simulink model "MultilayerProcessControlSim"  (R2023b)
settings: Solver=ode4  StartTime=0.0  StopTime=10  RelTol=1e-3
undefined symbols (not defined in the file): DiscIntNeverNeededParam
libraries: dspstat3 x22, slpidlib x14
(part 1 of 3)
settings Model: Creator=yagiz  LastModifiedBy=yagiz

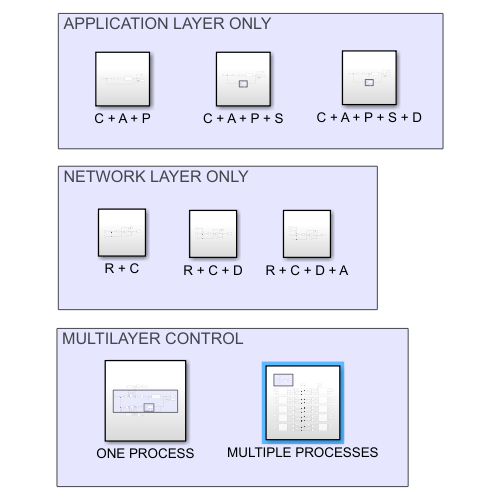
[thumbnail: Simulink's stored preview of the top-level diagram]
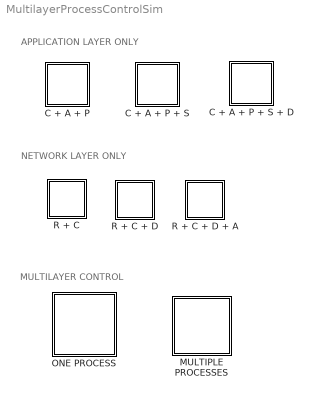
== system MultilayerProcessControlSim ==
  note: MULTILAYER CONTROL
  note: NETWORK LAYER ONLY
  note: APPLICATION LAYER ONLY
  C + A + P : Subsystem
  C + A + P + S : Subsystem
  C + A + P + S + D : Subsystem
  MULTIPLE PROCESSES : Subsystem
  ONE PROCESS : Subsystem
  R + C : Subsystem
  R + C + D : Subsystem
  R + C + D + A : Subsystem

== system MultilayerProcessControlSim/C + A + P ==
  ACTUATOR : Saturate  UpperLimit=150  LowerLimit=-150
  CONTROLLER : slpidlib/PID Controller  Controller=PI  Form=Parallel  TimeDomain=Continuous-time  UseExternalTs=off  SampleTime=-1  IntegratorMethod=Forward Euler  FilterMethod=Forward Euler  ControllerParametersSource=internal  P=1  I=3.6  UseKiTs=off  D=0  N=100  UseFilter=on  TunerSelectOption=Transfer Function Based (PID Tuner App)  InitialConditionSource=internal  InitialConditionForIntegrator=0  InitialConditionForFilter=0  DifferentiatorICPrevScaledInput=0  ExternalReset=none  TrackingMode=off  Kt=1  LimitOutput=off  SatLimitsSource=internal  UpperSaturationLimit=inf  LowerSaturationLimit=-inf  LinearizeAsGain=on  AntiWindupMode=none  Kb=1  LimitIntegrator=off  UpperIntegratorSaturationLimit=inf  LowerIntegratorSaturationLimit=-inf  POutMin=[]  POutMax=[]  IOutMin=[]  IOutMax=[]  DOutMin=[]  DOutMax=[]  NOutMin=[]  NOutMax=[]  SumOutMin=[]  SumOutMax=[]  SaturationOutMin=[]  SaturationOutMax=[]  PParamMin=[]  PParamMax=[]  IParamMin=[]  IParamMax=[]  DParamMin=[]  DParamMax=[]  NParamMin=[]  NParamMax=[]  KbParamMin=[]  KbParamMax=[]  KtParamMin=[]  KtParamMax=[]  KbOutMin=[]  KbOutMax=[]  KtOutMin=[]  KtOutMax=[]  IntegratorOutMin=[]  IntegratorOutMax=[]  FilterOutMin=[]  FilterOutMax=[]  SumI1OutMin=[]  SumI1OutMax=[]  SumI2OutMin=[]  SumI2OutMax=[]  SumI3OutMin=[]  SumI3OutMax=[]  SumI4OutMin=[]  SumI4OutMax=[]  SumDOutMin=[]  SumDOutMax=[]  DifferentiatorOutMin=[]  DifferentiatorOutMax=[]  FilterDiffOutCoefMin=[]  FilterDiffOutCoefMax=[]  ReciprocalOutMin=[]  ReciprocalOutMax=[]  SumDenOutMin=[]  SumDenOutMax=[]  SumNumOutMin=[]  SumNumOutMax=[]  DivideOutMin=[]  DivideOutMax=[]  UdiffTsProdOutMin=[]  UdiffTsProdOutMax=[]  NTsProdOutMin=[]  NTsProdOutMax=[]  UintegralTsProdOutMin=[]  UintegralTsProdOutMax=[]  UngainTsProdOutMin=[]  UngainTsProdOutMax=[]  ClampingZeroOutDataTypeStr=Inherit: Inherit via back propagation  ClampingZeroOutMin=[]  ClampingZeroOutMax=[]  FilterDenConstantOutDataTypeStr=Inherit: Inherit via back propagation  FilterDenConstantOutMin=[]  FilterDenConstantOutMax=[]  PCopyOutDataTypeStr=Inherit: Inherit via back propagation  PCopyOutMin=[]  PCopyOutMax=[]  NCopyOutDataTypeStr=Inherit: Inherit via back propagation  NCopyOutMin=[]  NCopyOutMax=[]  IntegratorContinuousStateAttributes=''  IntegratorStateMustResolveToSignalObject=off  IntegratorRTWStateStorageClass=Auto  FilterContinuousStateAttributes=''  FilterStateMustResolveToSignalObject=off  FilterRTWStateStorageClass=Auto  ParallelPVariant=InternalParameters  IdealPVariant=Disabled  IVariant=InternalParameters  DVariant=Disabled  IntegratorVariant=Continuous  SatVariant=Disabled  AWVariant=Passthrough  PCopyVariant=Disabled  TRVariant=Disabled  FdbkBlocksVariant=Forward  IdealPFdbkVariant=Disabled  SatFdbkVariant=Disabled  DerivativeFilterVariant=Disabled  NVariant=Disabled  NCopyVariant=Disabled_SignalSpec  FilterICVariant=Disabled  IntegratorICVariant=InternalICs  ExternalResetVariant=Disabled  TRSumVariant=Passthrough  SumFdbkVariant=Disabled  SumVariant=Sum_PI  TsampFilterVariant=InternalTs  TsampNgainVariant=Passthrough  TsampIntegralVariant=Disabled_SignalSpec  ExternalSaturationOutDataTypeStr=Inherit: Same as second input
  Constant3 : Constant  Value=20
  PROCESS : TransferFcn  Numerator=[1.38]  Denominator=[0.0007 0.1 0.00483]
  SETPOINT : Step  After=20  SampleTime=0
  Scope : Scope
  Sum : Sum  Inputs=|+-
  Sum4 : Sum  Inputs=|-+
  error : Display
  final value : Display
  wires:
  Sum/1 -> CONTROLLER/1
  CONTROLLER/1 -> ACTUATOR/1
  PROCESS/1 -> Sum4/1, Scope/1, final value/1, Sum/2  "output_app"
  Sum4/1 -> error/1
  SETPOINT/1 -> Sum/1
  Constant3/1 -> Sum4/2
  ACTUATOR/1 -> PROCESS/1

== system MultilayerProcessControlSim/C + A + P + S ==
  note: SENSOR
  ACTUATOR : Saturate  UpperLimit=150  LowerLimit=-150
  CONTROLLER : slpidlib/PID Controller  Controller=PI  Form=Parallel  TimeDomain=Continuous-time  UseExternalTs=off  SampleTime=-1  IntegratorMethod=Forward Euler  FilterMethod=Forward Euler  ControllerParametersSource=internal  P=1  I=3.6  UseKiTs=off  D=0  N=100  UseFilter=on  TunerSelectOption=Transfer Function Based (PID Tuner App)  InitialConditionSource=internal  InitialConditionForIntegrator=0  InitialConditionForFilter=0  DifferentiatorICPrevScaledInput=0  ExternalReset=none  TrackingMode=off  Kt=1  LimitOutput=off  SatLimitsSource=internal  UpperSaturationLimit=inf  LowerSaturationLimit=-inf  LinearizeAsGain=on  AntiWindupMode=none  Kb=1  LimitIntegrator=off  UpperIntegratorSaturationLimit=inf  LowerIntegratorSaturationLimit=-inf  POutMin=[]  POutMax=[]  IOutMin=[]  IOutMax=[]  DOutMin=[]  DOutMax=[]  NOutMin=[]  NOutMax=[]  SumOutMin=[]  SumOutMax=[]  SaturationOutMin=[]  SaturationOutMax=[]  PParamMin=[]  PParamMax=[]  IParamMin=[]  IParamMax=[]  DParamMin=[]  DParamMax=[]  NParamMin=[]  NParamMax=[]  KbParamMin=[]  KbParamMax=[]  KtParamMin=[]  KtParamMax=[]  KbOutMin=[]  KbOutMax=[]  KtOutMin=[]  KtOutMax=[]  IntegratorOutMin=[]  IntegratorOutMax=[]  FilterOutMin=[]  FilterOutMax=[]  SumI1OutMin=[]  SumI1OutMax=[]  SumI2OutMin=[]  SumI2OutMax=[]  SumI3OutMin=[]  SumI3OutMax=[]  SumI4OutMin=[]  SumI4OutMax=[]  SumDOutMin=[]  SumDOutMax=[]  DifferentiatorOutMin=[]  DifferentiatorOutMax=[]  FilterDiffOutCoefMin=[]  FilterDiffOutCoefMax=[]  ReciprocalOutMin=[]  ReciprocalOutMax=[]  SumDenOutMin=[]  SumDenOutMax=[]  SumNumOutMin=[]  SumNumOutMax=[]  DivideOutMin=[]  DivideOutMax=[]  UdiffTsProdOutMin=[]  UdiffTsProdOutMax=[]  NTsProdOutMin=[]  NTsProdOutMax=[]  UintegralTsProdOutMin=[]  UintegralTsProdOutMax=[]  UngainTsProdOutMin=[]  UngainTsProdOutMax=[]  ClampingZeroOutDataTypeStr=Inherit: Inherit via back propagation  ClampingZeroOutMin=[]  ClampingZeroOutMax=[]  FilterDenConstantOutDataTypeStr=Inherit: Inherit via back propagation  FilterDenConstantOutMin=[]  FilterDenConstantOutMax=[]  PCopyOutDataTypeStr=Inherit: Inherit via back propagation  PCopyOutMin=[]  PCopyOutMax=[]  NCopyOutDataTypeStr=Inherit: Inherit via back propagation  NCopyOutMin=[]  NCopyOutMax=[]  IntegratorContinuousStateAttributes=''  IntegratorStateMustResolveToSignalObject=off  IntegratorRTWStateStorageClass=Auto  FilterContinuousStateAttributes=''  FilterStateMustResolveToSignalObject=off  FilterRTWStateStorageClass=Auto  ParallelPVariant=InternalParameters  IdealPVariant=Disabled  IVariant=InternalParameters  DVariant=Disabled  IntegratorVariant=Continuous  SatVariant=Disabled  AWVariant=Passthrough  PCopyVariant=Disabled  TRVariant=Disabled  FdbkBlocksVariant=Forward  IdealPFdbkVariant=Disabled  SatFdbkVariant=Disabled  DerivativeFilterVariant=Disabled  NVariant=Disabled  NCopyVariant=Disabled_SignalSpec  FilterICVariant=Disabled  IntegratorICVariant=InternalICs  ExternalResetVariant=Disabled  TRSumVariant=Passthrough  SumFdbkVariant=Disabled  SumVariant=Sum_PI  TsampFilterVariant=InternalTs  TsampNgainVariant=Passthrough  TsampIntegralVariant=Disabled_SignalSpec  ExternalSaturationOutDataTypeStr=Inherit: Same as second input
  Constant3 : Constant  Value=20
  PROCESS : TransferFcn  Numerator=[1.38]  Denominator=[0.0007 0.1 0.00483]
  SETPOINT : Step  After=20  SampleTime=0
  Scope : Scope
  Sensor Accuracy : Sin  Amplitude=0.01  Bias=0.01  Frequency=50  SampleTime=0
  Sensor TF : TransferFcn  Denominator=[0.0002 1]
  Sum : Sum  Inputs=|+-
  Sum3 : Sum  Inputs=|++
  Sum4 : Sum  Inputs=|-+
  error : Display
  final value : Display
  wires:
  PROCESS/1 -> Sensor TF/1, Sum4/1, Scope/1, final value/1  "output_app"
  Sum/1 -> CONTROLLER/1
  CONTROLLER/1 -> ACTUATOR/1
  Constant3/1 -> Sum4/2
  Sum3/1 -> Sum/2
  ACTUATOR/1 -> PROCESS/1
  Sum4/1 -> error/1
  SETPOINT/1 -> Sum/1
  Sensor TF/1 -> Sum3/1
  Sensor Accuracy/1 -> Sum3/2

== system MultilayerProcessControlSim/C + A + P + S + D ==
  note: SENSOR
  ACTUATOR : Saturate  UpperLimit=150  LowerLimit=-150
  CONTROLLER : slpidlib/PID Controller  Controller=PI  Form=Parallel  TimeDomain=Continuous-time  UseExternalTs=off  SampleTime=-1  IntegratorMethod=Forward Euler  FilterMethod=Forward Euler  ControllerParametersSource=internal  P=1  I=3.6  UseKiTs=off  D=0  N=100  UseFilter=on  TunerSelectOption=Transfer Function Based (PID Tuner App)  InitialConditionSource=internal  InitialConditionForIntegrator=0  InitialConditionForFilter=0  DifferentiatorICPrevScaledInput=0  ExternalReset=none  TrackingMode=off  Kt=1  LimitOutput=off  SatLimitsSource=internal  UpperSaturationLimit=inf  LowerSaturationLimit=-inf  LinearizeAsGain=on  AntiWindupMode=none  Kb=1  LimitIntegrator=off  UpperIntegratorSaturationLimit=inf  LowerIntegratorSaturationLimit=-inf  POutMin=[]  POutMax=[]  IOutMin=[]  IOutMax=[]  DOutMin=[]  DOutMax=[]  NOutMin=[]  NOutMax=[]  SumOutMin=[]  SumOutMax=[]  SaturationOutMin=[]  SaturationOutMax=[]  PParamMin=[]  PParamMax=[]  IParamMin=[]  IParamMax=[]  DParamMin=[]  DParamMax=[]  NParamMin=[]  NParamMax=[]  KbParamMin=[]  KbParamMax=[]  KtParamMin=[]  KtParamMax=[]  KbOutMin=[]  KbOutMax=[]  KtOutMin=[]  KtOutMax=[]  IntegratorOutMin=[]  IntegratorOutMax=[]  FilterOutMin=[]  FilterOutMax=[]  SumI1OutMin=[]  SumI1OutMax=[]  SumI2OutMin=[]  SumI2OutMax=[]  SumI3OutMin=[]  SumI3OutMax=[]  SumI4OutMin=[]  SumI4OutMax=[]  SumDOutMin=[]  SumDOutMax=[]  DifferentiatorOutMin=[]  DifferentiatorOutMax=[]  FilterDiffOutCoefMin=[]  FilterDiffOutCoefMax=[]  ReciprocalOutMin=[]  ReciprocalOutMax=[]  SumDenOutMin=[]  SumDenOutMax=[]  SumNumOutMin=[]  SumNumOutMax=[]  DivideOutMin=[]  DivideOutMax=[]  UdiffTsProdOutMin=[]  UdiffTsProdOutMax=[]  NTsProdOutMin=[]  NTsProdOutMax=[]  UintegralTsProdOutMin=[]  UintegralTsProdOutMax=[]  UngainTsProdOutMin=[]  UngainTsProdOutMax=[]  ClampingZeroOutDataTypeStr=Inherit: Inherit via back propagation  ClampingZeroOutMin=[]  ClampingZeroOutMax=[]  FilterDenConstantOutDataTypeStr=Inherit: Inherit via back propagation  FilterDenConstantOutMin=[]  FilterDenConstantOutMax=[]  PCopyOutDataTypeStr=Inherit: Inherit via back propagation  PCopyOutMin=[]  PCopyOutMax=[]  NCopyOutDataTypeStr=Inherit: Inherit via back propagation  NCopyOutMin=[]  NCopyOutMax=[]  IntegratorContinuousStateAttributes=''  IntegratorStateMustResolveToSignalObject=off  IntegratorRTWStateStorageClass=Auto  FilterContinuousStateAttributes=''  FilterStateMustResolveToSignalObject=off  FilterRTWStateStorageClass=Auto  ParallelPVariant=InternalParameters  IdealPVariant=Disabled  IVariant=InternalParameters  DVariant=Disabled  IntegratorVariant=Continuous  SatVariant=Disabled  AWVariant=Passthrough  PCopyVariant=Disabled  TRVariant=Disabled  FdbkBlocksVariant=Forward  IdealPFdbkVariant=Disabled  SatFdbkVariant=Disabled  DerivativeFilterVariant=Disabled  NVariant=Disabled  NCopyVariant=Disabled_SignalSpec  FilterICVariant=Disabled  IntegratorICVariant=InternalICs  ExternalResetVariant=Disabled  TRSumVariant=Passthrough  SumFdbkVariant=Disabled  SumVariant=Sum_PI  TsampFilterVariant=InternalTs  TsampNgainVariant=Passthrough  TsampIntegralVariant=Disabled_SignalSpec  ExternalSaturationOutDataTypeStr=Inherit: Same as second input
  Constant3 : Constant  Value=20
  DISTURBANCE : Sin  Amplitude=0.1  Bias=0.1  Frequency=50  SampleTime=0
  PROCESS : TransferFcn  Numerator=[1.38]  Denominator=[0.0007 0.1 0.00483]
  SETPOINT : Step  After=20  SampleTime=0
  Scope : Scope
  Sensor Accuracy : Sin  Amplitude=0.01  Frequency=50  SampleTime=0
  Sensor TF : TransferFcn  Denominator=[0.0002 1]
  Sum : Sum  Inputs=|+-
  Sum2 : Sum  Inputs=|++
  Sum3 : Sum  Inputs=|++
  Sum4 : Sum  Inputs=|-+
  error : Display
  final value : Display
  wires:
  PROCESS/1 -> Sensor TF/1, Sum4/1, Scope/1, final value/1  "output_app"
  Sensor TF/1 -> Sum3/1
  Sensor Accuracy/1 -> Sum3/2
  Sum3/1 -> Sum/2
  CONTROLLER/1 -> ACTUATOR/1
  SETPOINT/1 -> Sum/1
  Sum4/1 -> error/1
  Constant3/1 -> Sum4/2
  Sum/1 -> CONTROLLER/1
  DISTURBANCE/1 -> Sum2/2
  ACTUATOR/1 -> Sum2/1
  Sum2/1 -> PROCESS/1

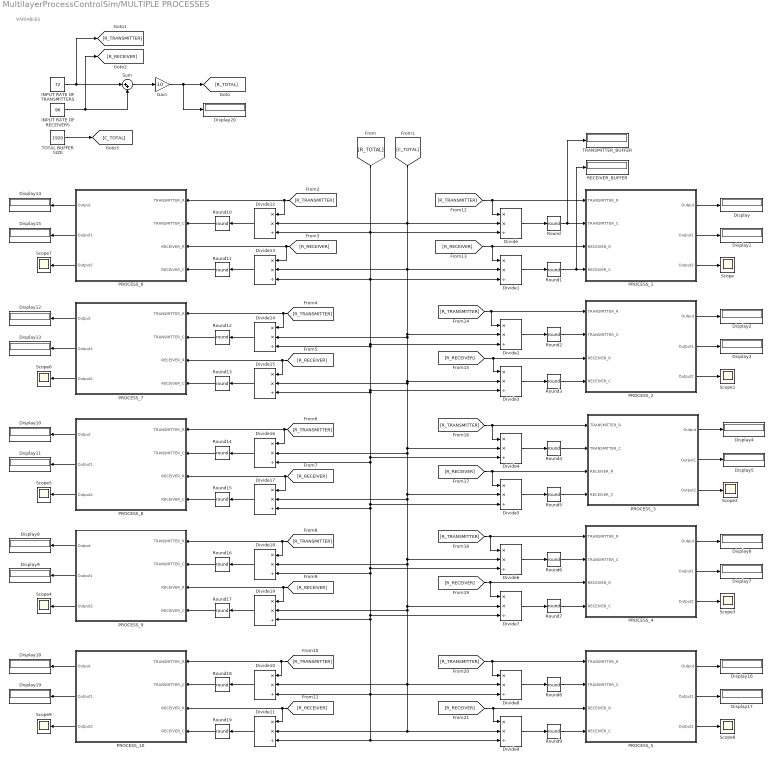
== system MultilayerProcessControlSim/MULTIPLE PROCESSES ==
  note: VARIABLES
  Display{,1..20} (21 alike) : Display
  Divide{,1..19} (20 alike) : Product  Inputs=**/
  Gain : Gain  Gain=10
  INPUT RATE OF RECEIVERS : Constant  Value=96
  INPUT RATE OF TRANSMITTERS : Constant  Value=72
  PROCESS_1 : Subsystem
  PROCESS_10 : Subsystem
  PROCESS_2 : Subsystem
  PROCESS_3 : Subsystem
  PROCESS_4 : Subsystem
  PROCESS_5 : Subsystem
  PROCESS_6 : Subsystem
  PROCESS_7 : Subsystem
  PROCESS_8 : Subsystem
  PROCESS_9 : Subsystem
  RECEIVER_BUFFER : Display
  Round{,1..19} (20 alike) : Rounding  Operator=round
  Scope{,1..9} (10 alike) : Scope
  Sum : Sum  Inputs=|++
  TOTAL BUFFER SIZE : Constant  Value=1920
  TRANSMITTER_BUFFER : Display
  wires:
  [C_TOTAL] -> Divide12/2, Divide13/2, Divide14/2, Divide15/2, Divide16/2, Divide17/2, Divide18/2, Divide19/2, Divide10/2, Divide8/2, Divide9/2, Divide11/2, Divide7/2, Divide6/2, Divide5/2, Divide4/2, Divide3/2, Divide2/2, Divide1/2, Divide/2
  Round2/1 -> PROCESS_2/2(TRANSMITTER_C)
  Round4/1 -> PROCESS_3/2(TRANSMITTER_C)
  [R_RECEIVER] -> Divide11/1, PROCESS_10/3(RECEIVER_R)
  Round17/1 -> PROCESS_9/4(RECEIVER_C)
  Round11/1 -> PROCESS_6/4(RECEIVER_C)
  PROCESS_5/2(Output1) -> Display17/1
  Divide6/1 -> Round6/1
  [R_TOTAL] -> Divide12/3, Divide13/3, Divide2/3, Divide14/3, Divide15/3, Divide16/3, Divide5/3, Divide17/3, Divide18/3, Divide19/3, Divide10/3, Divide11/3, Divide9/3, Divide8/3, Divide7/3, Divide6/3, Divide4/3, Divide3/3, Divide1/3, Divide/3
  Round12/1 -> PROCESS_7/2(TRANSMITTER_C)
  [R_RECEIVER] -> Divide1/1, PROCESS_1/3(RECEIVER_R)
  Round14/1 -> PROCESS_8/2(TRANSMITTER_C)
  Round10/1 -> PROCESS_6/2(TRANSMITTER_C)
  [R_TRANSMITTER] -> Divide10/1, PROCESS_10/1(TRANSMITTER_R)
  [R_RECEIVER] -> Divide13/1, PROCESS_6/3(RECEIVER_R)
  Divide17/1 -> Round15/1
  Divide11/1 -> Round19/1
  PROCESS_2/2(Output1) -> Display3/1
  [R_TRANSMITTER] -> Divide12/1, PROCESS_6/1(TRANSMITTER_R)
  PROCESS_6/1(Output) -> Display14/1
  Round3/1 -> PROCESS_2/4(RECEIVER_C)
  [R_RECEIVER] -> Divide5/1, PROCESS_3/3(RECEIVER_R)
  Round13/1 -> PROCESS_7/4(RECEIVER_C)
  Divide/1 -> Round/1
  [R_TRANSMITTER] -> Divide4/1, PROCESS_3/1(TRANSMITTER_R)
  [R_RECEIVER] -> Divide9/1, PROCESS_5/3(RECEIVER_R)
  Divide13/1 -> Round11/1
  PROCESS_2/3(Output2) -> Scope1/1
  [R_TRANSMITTER] -> Divide14/1, PROCESS_7/1(TRANSMITTER_R)
  [R_RECEIVER] -> Divide15/1, PROCESS_7/3(RECEIVER_R)
  PROCESS_10/1(Output) -> Display18/1
  [R_TRANSMITTER] -> Divide2/1, PROCESS_2/1(TRANSMITTER_R)
  Divide4/1 -> Round4/1
  PROCESS_1/1(Output) -> Display/1
  Round19/1 -> PROCESS_10/4(RECEIVER_C)
  PROCESS_9/1(Output) -> Display8/1
  PROCESS_2/1(Output) -> Display2/1
  PROCESS_10/3(Output2) -> Scope9/1
  Round9/1 -> PROCESS_5/4(RECEIVER_C)
  [R_TRANSMITTER] -> Divide6/1, PROCESS_4/1(TRANSMITTER_R)
  Divide9/1 -> Round9/1
  Round5/1 -> PROCESS_3/4(RECEIVER_C)
  PROCESS_10/2(Output1) -> Display19/1
  INPUT RATE OF TRANSMITTERS/1 -> [R_TRANSMITTER], Sum/1
  [R_TRANSMITTER] -> Divide8/1, PROCESS_5/1(TRANSMITTER_R)
  [R_RECEIVER] -> Divide17/1, PROCESS_8/3(RECEIVER_R)
  PROCESS_7/2(Output1) -> Display13/1
  Divide12/1 -> Round10/1
  Sum/1 -> Gain/1
  [R_TRANSMITTER] -> Divide18/1, PROCESS_9/1(TRANSMITTER_R)
  [R_TRANSMITTER] -> Divide16/1, PROCESS_8/1(TRANSMITTER_R)
  INPUT RATE OF RECEIVERS/1 -> Sum/2, [R_RECEIVER]
  [R_RECEIVER] -> Divide19/1, PROCESS_9/3(RECEIVER_R)
  PROCESS_5/1(Output) -> Display16/1
  Divide14/1 -> Round12/1
  PROCESS_7/1(Output) -> Display12/1
  PROCESS_3/3(Output2) -> Scope2/1
  Divide1/1 -> Round1/1
  Divide2/1 -> Round2/1
  Round15/1 -> PROCESS_8/4(RECEIVER_C)
  Divide3/1 -> Round3/1
  [R_RECEIVER] -> Divide3/1, PROCESS_2/3(RECEIVER_R)
  Round1/1 -> RECEIVER_BUFFER/1, PROCESS_1/4(RECEIVER_C)
  Divide19/1 -> Round17/1
  PROCESS_4/2(Output1) -> Display7/1
  Round18/1 -> PROCESS_10/2(TRANSMITTER_C)
  Gain/1 -> [R_TOTAL], Display20/1
  PROCESS_5/3(Output2) -> Scope8/1
  [R_TRANSMITTER] -> Divide/1, PROCESS_1/1(TRANSMITTER_R)
  PROCESS_1/3(Output2) -> Scope/1
  [R_RECEIVER] -> Divide7/1, PROCESS_4/3(RECEIVER_R)
  Divide10/1 -> Round18/1
  PROCESS_1/2(Output1) -> Display1/1
  PROCESS_4/1(Output) -> Display6/1
  Round16/1 -> PROCESS_9/2(TRANSMITTER_C)
  PROCESS_8/2(Output1) -> Display11/1
  Round/1 -> TRANSMITTER_BUFFER/1, PROCESS_1/2(TRANSMITTER_C)
  Round8/1 -> PROCESS_5/2(TRANSMITTER_C)
  PROCESS_7/3(Output2) -> Scope6/1
  PROCESS_6/3(Output2) -> Scope7/1
  PROCESS_6/2(Output1) -> Display15/1
  PROCESS_8/1(Output) -> Display10/1
  PROCESS_8/3(Output2) -> Scope5/1
  PROCESS_9/3(Output2) -> Scope4/1
  PROCESS_9/2(Output1) -> Display9/1
  Divide18/1 -> Round16/1
  PROCESS_3/2(Output1) -> Display5/1
  PROCESS_3/1(Output) -> Display4/1
  PROCESS_4/3(Output2) -> Scope3/1
  TOTAL BUFFER SIZE/1 -> [C_TOTAL]
  Round6/1 -> PROCESS_4/2(TRANSMITTER_C)
  Round7/1 -> PROCESS_4/4(RECEIVER_C)
  Divide7/1 -> Round7/1
  Divide5/1 -> Round5/1
  Divide16/1 -> Round14/1
  Divide8/1 -> Round8/1
  Divide15/1 -> Round13/1

== system MultilayerProcessControlSim/ONE PROCESS ==
  note: APPLICATION LAYER
  note: SENSOR
  ACTUATOR : Saturate  UpperLimit=150  LowerLimit=-150
  AVERAGE DELAY1 : Display
  AVERAGE DELAY2 : Display
  CONTROLLER : slpidlib/PID Controller  Controller=PI  Form=Parallel  TimeDomain=Continuous-time  UseExternalTs=off  SampleTime=-1  IntegratorMethod=Forward Euler  FilterMethod=Forward Euler  ControllerParametersSource=internal  P=1  I=3.6  UseKiTs=off  D=0  N=100  UseFilter=on  TunerSelectOption=Transfer Function Based (PID Tuner App)  InitialConditionSource=internal  InitialConditionForIntegrator=0  InitialConditionForFilter=0  DifferentiatorICPrevScaledInput=0  ExternalReset=none  TrackingMode=off  Kt=1  LimitOutput=off  SatLimitsSource=internal  UpperSaturationLimit=inf  LowerSaturationLimit=-inf  LinearizeAsGain=on  AntiWindupMode=none  Kb=1  LimitIntegrator=off  UpperIntegratorSaturationLimit=inf  LowerIntegratorSaturationLimit=-inf  POutMin=[]  POutMax=[]  IOutMin=[]  IOutMax=[]  DOutMin=[]  DOutMax=[]  NOutMin=[]  NOutMax=[]  SumOutMin=[]  SumOutMax=[]  SaturationOutMin=[]  SaturationOutMax=[]  PParamMin=[]  PParamMax=[]  IParamMin=[]  IParamMax=[]  DParamMin=[]  DParamMax=[]  NParamMin=[]  NParamMax=[]  KbParamMin=[]  KbParamMax=[]  KtParamMin=[]  KtParamMax=[]  KbOutMin=[]  KbOutMax=[]  KtOutMin=[]  KtOutMax=[]  IntegratorOutMin=[]  IntegratorOutMax=[]  FilterOutMin=[]  FilterOutMax=[]  SumI1OutMin=[]  SumI1OutMax=[]  SumI2OutMin=[]  SumI2OutMax=[]  SumI3OutMin=[]  SumI3OutMax=[]  SumI4OutMin=[]  SumI4OutMax=[]  SumDOutMin=[]  SumDOutMax=[]  DifferentiatorOutMin=[]  DifferentiatorOutMax=[]  FilterDiffOutCoefMin=[]  FilterDiffOutCoefMax=[]  ReciprocalOutMin=[]  ReciprocalOutMax=[]  SumDenOutMin=[]  SumDenOutMax=[]  SumNumOutMin=[]  SumNumOutMax=[]  DivideOutMin=[]  DivideOutMax=[]  UdiffTsProdOutMin=[]  UdiffTsProdOutMax=[]  NTsProdOutMin=[]  NTsProdOutMax=[]  UintegralTsProdOutMin=[]  UintegralTsProdOutMax=[]  UngainTsProdOutMin=[]  UngainTsProdOutMax=[]  ClampingZeroOutDataTypeStr=Inherit: Inherit via back propagation  ClampingZeroOutMin=[]  ClampingZeroOutMax=[]  FilterDenConstantOutDataTypeStr=Inherit: Inherit via back propagation  FilterDenConstantOutMin=[]  FilterDenConstantOutMax=[]  PCopyOutDataTypeStr=Inherit: Inherit via back propagation  PCopyOutMin=[]  PCopyOutMax=[]  NCopyOutDataTypeStr=Inherit: Inherit via back propagation  NCopyOutMin=[]  NCopyOutMax=[]  IntegratorContinuousStateAttributes=''  IntegratorStateMustResolveToSignalObject=off  IntegratorRTWStateStorageClass=Auto  FilterContinuousStateAttributes=''  FilterStateMustResolveToSignalObject=off  FilterRTWStateStorageClass=Auto  ParallelPVariant=InternalParameters  IdealPVariant=Disabled  IVariant=InternalParameters  DVariant=Disabled  IntegratorVariant=Continuous  SatVariant=Disabled  AWVariant=Passthrough  PCopyVariant=Disabled  TRVariant=Disabled  FdbkBlocksVariant=Forward  IdealPFdbkVariant=Disabled  SatFdbkVariant=Disabled  DerivativeFilterVariant=Disabled  NVariant=Disabled  NCopyVariant=Disabled_SignalSpec  FilterICVariant=Disabled  IntegratorICVariant=InternalICs  ExternalResetVariant=Disabled  TRSumVariant=Passthrough  SumFdbkVariant=Disabled  SumVariant=Sum_PI  TsampFilterVariant=InternalTs  TsampNgainVariant=Passthrough  TsampIntegralVariant=Disabled_SignalSpec  ExternalSaturationOutDataTypeStr=Inherit: Same as second input
  Constant3 : Constant  Value=20
  DISTURBANCE : Sin  Amplitude=0.1  Bias=0.05  Frequency=50  SampleTime=0
  DRIVER-PLC NETWORK : Subsystem
  Memory : Memory
  Memory1 : Memory
  Moving Average : dspstat3/Moving Average  Method=Sliding window  ForgettingFactorPort=off  SpecifyWindowLength=on  WindowLength=4  OverlapLength=3  AllowArbitraryInputLength=off  ForgettingFactor=0.9  SimulateUsing=Code generation
  Moving Average1 : dspstat3/Moving Average  Method=Sliding window  ForgettingFactorPort=off  SpecifyWindowLength=on  WindowLength=4  OverlapLength=3  AllowArbitraryInputLength=off  ForgettingFactor=0.9  SimulateUsing=Code generation
  PLC-DRIVER NETWORK : Subsystem
  PROCESS : TransferFcn  Numerator=[1.38]  Denominator=[0.0007 0.1 0.00483]
  SETPOINT : Step  After=20  SampleTime=0
  Scope1 : Scope  NumInputPorts=2
  Sensor Accuracy : Sin  Amplitude=0.01  Frequency=50  SampleTime=0
  Sensor TF : TransferFcn  Denominator=[0.0002 1]
  Sum : Sum  Inputs=|+-
  Sum2 : Sum  Inputs=|++
  Sum3 : Sum  Inputs=|++
  Sum4 : Sum  Inputs=|-+
  Switch : Switch  Criteria=u2 > Threshold  Threshold=9600  SaturateOnIntegerOverflow=off  InputSameDT=off
  Switch1 : Switch  Criteria=u2 > Threshold  Threshold=9600  SaturateOnIntegerOverflow=off  InputSameDT=off
  Variable Time Delay : VariableTransportDelay  MaximumDelay=10
  Variable Time Delay1 : VariableTransportDelay  MaximumDelay=10
  error : Display
  final value : Display
  wires:
  Moving Average1/1 -> AVERAGE DELAY1/1
  Sum2/1 -> PROCESS/1
  Moving Average/1 -> AVERAGE DELAY2/1
  Switch1/1 -> Memory1/1, Variable Time Delay1/1
  Variable Time Delay/1 -> ACTUATOR/1
  DRIVER-PLC NETWORK/2(DELAY1) -> Variable Time Delay1/2, Moving Average/1
  Sum/1 -> CONTROLLER/1
  PROCESS/1 -> final value/1, Sum4/1, Scope1/2, Sensor TF/1  "output_app"
  DRIVER-PLC NETWORK/1(Q) -> Switch1/2
  PLC-DRIVER NETWORK/1(DELAY1) -> Moving Average1/1, Variable Time Delay/2
  SETPOINT/1 -> Sum/1
  PLC-DRIVER NETWORK/2(Q) -> Switch/2
  Sensor TF/1 -> Sum3/1
  Constant3/1 -> Sum4/2
  Sensor Accuracy/1 -> Sum3/2
  Sum4/1 -> error/1
  Switch/1 -> Memory/1, Variable Time Delay/1
  Variable Time Delay1/1 -> Sum/2, Scope1/1  "feedback_out"
  CONTROLLER/1 -> Switch/3
  Memory1/1 -> Switch1/1
  DISTURBANCE/1 -> Sum2/2
  ACTUATOR/1 -> Sum2/1
  Memory/1 -> Switch/1
  Sum3/1 -> Switch1/3

== system MultilayerProcessControlSim/R + C ==
  BUFFER : Constant  Value=96
  Discrete-Time Integrator1 : DiscreteIntegrator  SampleTime=-1  LimitOutput=on  UpperSaturationLimit=9600  LowerSaturationLimit=0  ICPrevOutput=DiscIntNeverNeededParam  ICPrevScaledInput=DiscIntNeverNeededParam
  Divide1 : Product  Inputs=*/
  INPUT RATE : Constant  Value=72
  Network Delay : Display
  PROPAGATION DELAY : Constant  Value=0.01
  Scope : Scope  NumInputPorts=2
  Sum1 : Sum  Inputs=|++
  Sum2 : Sum  Inputs=|+-
  wires:
  PROPAGATION DELAY/1 -> Sum1/2  "TAU_P"
  BUFFER/1 -> Divide1/2, Sum2/2
  Divide1/1 -> Sum1/1, Scope/2  "TAU_Q"
  Discrete-Time Integrator1/1 -> Scope/1, Divide1/1  "Q"
  INPUT RATE/1 -> Sum2/1
  Sum1/1 -> Network Delay/1  "DELAY"
  Sum2/1 -> Discrete-Time Integrator1/1  "Q_dot"

== system MultilayerProcessControlSim/R + C + D ==
  BUFFER : Constant  Value=96
  DISTURBANCE : DiscretePulseGenerator  PulseType=Time based  Amplitude=48  Period=0.01  PulseWidth=50
  Discrete-Time Integrator1 : DiscreteIntegrator  SampleTime=-1  LimitOutput=on  UpperSaturationLimit=9600  LowerSaturationLimit=0  ICPrevOutput=DiscIntNeverNeededParam  ICPrevScaledInput=DiscIntNeverNeededParam
  Divide1 : Product  Inputs=*/
  INPUT RATE : Constant  Value=72
  Network Delay : Display
  PROPAGATION DELAY : Constant  Value=0.01
  Scope : Scope  NumInputPorts=2
  Sum : Sum  Inputs=+|+|-
  Sum1 : Sum  Inputs=|++
  wires:
  BUFFER/1 -> Sum/3, Divide1/2
  Divide1/1 -> Sum1/1, Scope/2  "TAU_Q"
  INPUT RATE/1 -> Sum/2
  DISTURBANCE/1 -> Sum/1
  Sum1/1 -> Network Delay/1  "DELAY"
  PROPAGATION DELAY/1 -> Sum1/2  "TAU_P"
  Discrete-Time Integrator1/1 -> Scope/1, Divide1/1  "Q"
  Sum/1 -> Discrete-Time Integrator1/1  "Q_dot"

== system MultilayerProcessControlSim/R + C + D + A ==
  ATTACK : Constant  Value=10000
  BUFFER : Constant  Value=96
  DISTURBANCE : DiscretePulseGenerator  PulseType=Time based  Amplitude=24  Period=0.001  PulseWidth=50
  Discrete-Time Integrator1 : DiscreteIntegrator  SampleTime=-1  LimitOutput=on  UpperSaturationLimit=9600  LowerSaturationLimit=0  ICPrevOutput=DiscIntNeverNeededParam  ICPrevScaledInput=DiscIntNeverNeededParam
  Divide1 : Product  Inputs=*/
  INPUT RATE : Constant  Value=72
  Network Delay : Display
  PROPAGATION DELAY : Constant  Value=0.01
  Scope : Scope  NumInputPorts=2
  Sum : Sum  Inputs=++|+|-
  Sum1 : Sum  Inputs=|++
  wires:
  Divide1/1 -> Sum1/1, Scope/2  "TAU_Q"
  PROPAGATION DELAY/1 -> Sum1/2  "TAU_P"
  Sum1/1 -> Network Delay/1  "DELAY"
  Sum/1 -> Discrete-Time Integrator1/1  "Q_dot"
  Discrete-Time Integrator1/1 -> Scope/1, Divide1/1  "Q"
  BUFFER/1 -> Sum/4, Divide1/2
  INPUT RATE/1 -> Sum/3
  DISTURBANCE/1 -> Sum/2
  ATTACK/1 -> Sum/1

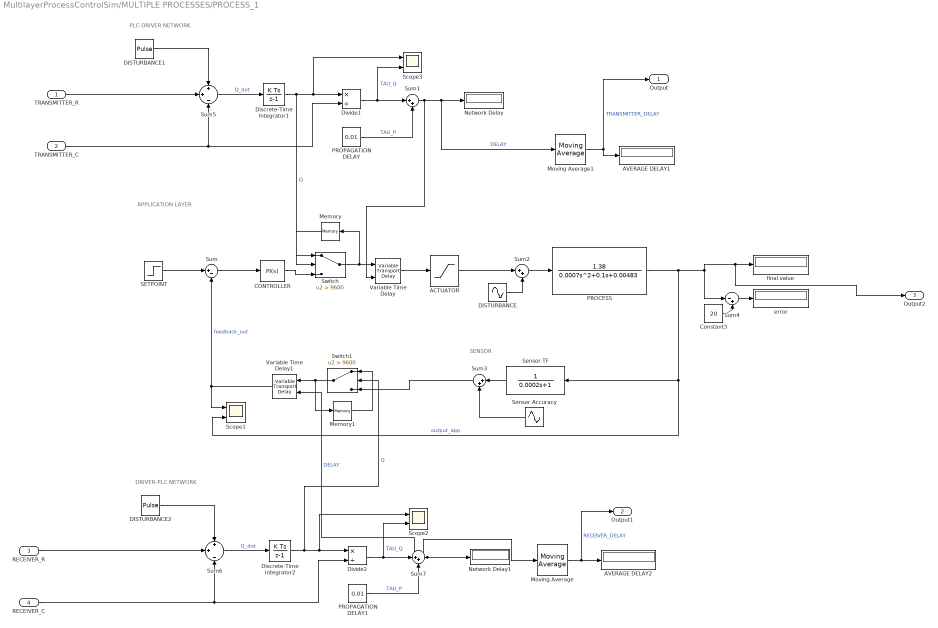
== system MultilayerProcessControlSim/MULTIPLE PROCESSES/PROCESS_1 ==
  note: DRIVER-PLC NETWORK
  note: PLC-DRIVER NETWORK
  note: APPLICATION LAYER
  note: SENSOR
  TRANSMITTER_R : Inport
  TRANSMITTER_C : Inport  Port=2
  RECEIVER_R : Inport  Port=3
  RECEIVER_C : Inport  Port=4
  ACTUATOR : Saturate  UpperLimit=150  LowerLimit=-150
  AVERAGE DELAY1 : Display
  AVERAGE DELAY2 : Display
  CONTROLLER : slpidlib/PID Controller  Controller=PI  Form=Parallel  TimeDomain=Continuous-time  UseExternalTs=off  SampleTime=-1  IntegratorMethod=Forward Euler  FilterMethod=Forward Euler  ControllerParametersSource=internal  P=1  I=3.6  UseKiTs=off  D=0  N=100  UseFilter=on  TunerSelectOption=Transfer Function Based (PID Tuner App)  InitialConditionSource=internal  InitialConditionForIntegrator=0  InitialConditionForFilter=0  DifferentiatorICPrevScaledInput=0  ExternalReset=none  TrackingMode=off  Kt=1  LimitOutput=off  SatLimitsSource=internal  UpperSaturationLimit=inf  LowerSaturationLimit=-inf  LinearizeAsGain=on  AntiWindupMode=none  Kb=1  LimitIntegrator=off  UpperIntegratorSaturationLimit=inf  LowerIntegratorSaturationLimit=-inf  POutMin=[]  POutMax=[]  IOutMin=[]  IOutMax=[]  DOutMin=[]  DOutMax=[]  NOutMin=[]  NOutMax=[]  SumOutMin=[]  SumOutMax=[]  SaturationOutMin=[]  SaturationOutMax=[]  PParamMin=[]  PParamMax=[]  IParamMin=[]  IParamMax=[]  DParamMin=[]  DParamMax=[]  NParamMin=[]  NParamMax=[]  KbParamMin=[]  KbParamMax=[]  KtParamMin=[]  KtParamMax=[]  KbOutMin=[]  KbOutMax=[]  KtOutMin=[]  KtOutMax=[]  IntegratorOutMin=[]  IntegratorOutMax=[]  FilterOutMin=[]  FilterOutMax=[]  SumI1OutMin=[]  SumI1OutMax=[]  SumI2OutMin=[]  SumI2OutMax=[]  SumI3OutMin=[]  SumI3OutMax=[]  SumI4OutMin=[]  SumI4OutMax=[]  SumDOutMin=[]  SumDOutMax=[]  DifferentiatorOutMin=[]  DifferentiatorOutMax=[]  FilterDiffOutCoefMin=[]  FilterDiffOutCoefMax=[]  ReciprocalOutMin=[]  ReciprocalOutMax=[]  SumDenOutMin=[]  SumDenOutMax=[]  SumNumOutMin=[]  SumNumOutMax=[]  DivideOutMin=[]  DivideOutMax=[]  UdiffTsProdOutMin=[]  UdiffTsProdOutMax=[]  NTsProdOutMin=[]  NTsProdOutMax=[]  UintegralTsProdOutMin=[]  UintegralTsProdOutMax=[]  UngainTsProdOutMin=[]  UngainTsProdOutMax=[]  ClampingZeroOutDataTypeStr=Inherit: Inherit via back propagation  ClampingZeroOutMin=[]  ClampingZeroOutMax=[]  FilterDenConstantOutDataTypeStr=Inherit: Inherit via back propagation  FilterDenConstantOutMin=[]  FilterDenConstantOutMax=[]  PCopyOutDataTypeStr=Inherit: Inherit via back propagation  PCopyOutMin=[]  PCopyOutMax=[]  NCopyOutDataTypeStr=Inherit: Inherit via back propagation  NCopyOutMin=[]  NCopyOutMax=[]  IntegratorContinuousStateAttributes=''  IntegratorStateMustResolveToSignalObject=off  IntegratorRTWStateStorageClass=Auto  FilterContinuousStateAttributes=''  FilterStateMustResolveToSignalObject=off  FilterRTWStateStorageClass=Auto  ParallelPVariant=InternalParameters  IdealPVariant=Disabled  IVariant=InternalParameters  DVariant=Disabled  IntegratorVariant=Continuous  SatVariant=Disabled  AWVariant=Passthrough  PCopyVariant=Disabled  TRVariant=Disabled  FdbkBlocksVariant=Forward  IdealPFdbkVariant=Disabled  SatFdbkVariant=Disabled  DerivativeFilterVariant=Disabled  NVariant=Disabled  NCopyVariant=Disabled_SignalSpec  FilterICVariant=Disabled  IntegratorICVariant=InternalICs  ExternalResetVariant=Disabled  TRSumVariant=Passthrough  SumFdbkVariant=Disabled  SumVariant=Sum_PI  TsampFilterVariant=InternalTs  TsampNgainVariant=Passthrough  TsampIntegralVariant=Disabled_SignalSpec  ExternalSaturationOutDataTypeStr=Inherit: Same as second input
  Constant3 : Constant  Value=20
  DISTURBANCE : Sin  Amplitude=0.1  Bias=0.05  Frequency=50  SampleTime=0
  DISTURBANCE1 : DiscretePulseGenerator  PulseType=Time based  Amplitude=0  Period=0.001  PulseWidth=50
  DISTURBANCE2 : DiscretePulseGenerator  PulseType=Time based  Amplitude=0  Period=0.001  PulseWidth=50
  Discrete-Time Integrator1 : DiscreteIntegrator  SampleTime=-1  LimitOutput=on  UpperSaturationLimit=9600  LowerSaturationLimit=0  ICPrevOutput=DiscIntNeverNeededParam  ICPrevScaledInput=DiscIntNeverNeededParam
  Discrete-Time Integrator2 : DiscreteIntegrator  SampleTime=-1  LimitOutput=on  UpperSaturationLimit=9600  LowerSaturationLimit=0  ICPrevOutput=DiscIntNeverNeededParam  ICPrevScaledInput=DiscIntNeverNeededParam
  Divide1 : Product  Inputs=*/
  Divide2 : Product  Inputs=*/
  Memory : Memory
  Memory1 : Memory
  Moving Average : dspstat3/Moving Average  Method=Sliding window  ForgettingFactorPort=off  SpecifyWindowLength=on  WindowLength=4  OverlapLength=3  AllowArbitraryInputLength=off  ForgettingFactor=0.9  SimulateUsing=Code generation
  Moving Average1 : dspstat3/Moving Average  Method=Sliding window  ForgettingFactorPort=off  SpecifyWindowLength=on  WindowLength=4  OverlapLength=3  AllowArbitraryInputLength=off  ForgettingFactor=0.9  SimulateUsing=Code generation
  Network Delay : Display
  Network Delay1 : Display
  PROCESS : TransferFcn  Numerator=[1.38]  Denominator=[0.0007 0.1 0.00483]
  PROPAGATION DELAY : Constant  Value=0.01
  PROPAGATION DELAY1 : Constant  Value=0.01
  SETPOINT : Step  After=20  SampleTime=0
  Scope1 : Scope  NumInputPorts=2
  Scope2 : Scope  NumInputPorts=2
  Scope3 : Scope  NumInputPorts=2
  Sensor Accuracy : Sin  Amplitude=0.01  Frequency=50  SampleTime=0
  Sensor TF : TransferFcn  Denominator=[0.0002 1]
  Sum : Sum  Inputs=|+-
  Sum{1..3,7} (4 alike) : Sum  Inputs=|++
  Sum4 : Sum  Inputs=|-+
  Sum5 : Sum  Inputs=+|+|-
  Sum6 : Sum  Inputs=+|+|-
  Switch : Switch  Criteria=u2 > Threshold  Threshold=9600  SaturateOnIntegerOverflow=off  InputSameDT=off
  Switch1 : Switch  Criteria=u2 > Threshold  Threshold=9600  SaturateOnIntegerOverflow=off  InputSameDT=off
  Variable Time Delay : VariableTransportDelay  MaximumDelay=10
  Variable Time Delay1 : VariableTransportDelay  MaximumDelay=10
  error : Display
  final value : Display
  Output : Outport
  Output1 : Outport  Port=2
  Output2 : Outport  Port=3
  wires:
  RECEIVER_C/1 -> Sum6/3, Divide2/2
  DISTURBANCE1/1 -> Sum5/1
  Sum1/1 -> Moving Average1/1, Network Delay/1, Variable Time Delay/2  "DELAY"
  TRANSMITTER_C/1 -> Divide1/2, Sum5/3
  CONTROLLER/1 -> Switch/3
  Sum3/1 -> Switch1/3
  Moving Average1/1 -> Output/1, AVERAGE DELAY1/1  "TRANSMITTER_DELAY"
  Memory1/1 -> Switch1/1
  Memory/1 -> Switch/1
  Switch/1 -> Memory/1, Variable Time Delay/1
  TRANSMITTER_R/1 -> Sum5/2
  ACTUATOR/1 -> Sum2/1
  RECEIVER_R/1 -> Sum6/2
  SETPOINT/1 -> Sum/1
  Sum7/1 -> Variable Time Delay1/2, Moving Average/1, Network Delay1/1  "DELAY"
  Discrete-Time Integrator2/1 -> Switch1/2, Scope2/1, Divide2/1  "Q"
  Switch1/1 -> Memory1/1, Variable Time Delay1/1
  DISTURBANCE2/1 -> Sum6/1
  Variable Time Delay1/1 -> Sum/2, Scope1/1  "feedback_out"
  Discrete-Time Integrator1/1 -> Scope3/1, Divide1/1, Switch/2  "Q"
  Divide2/1 -> Sum7/1, Scope2/2  "TAU_Q"
  Moving Average/1 -> Output1/1, AVERAGE DELAY2/1  "RECEIVER_DELAY"
  Divide1/1 -> Scope3/2, Sum1/1  "TAU_Q"
  Sensor Accuracy/1 -> Sum3/2
  Sum6/1 -> Discrete-Time Integrator2/1  "Q_dot"
  PROCESS/1 -> Output2/1, final value/1, Sum4/1, Sensor TF/1, Scope1/2  "output_app"
  PROPAGATION DELAY1/1 -> Sum7/2  "TAU_P"
  Sum5/1 -> Discrete-Time Integrator1/1  "Q_dot"
  Sum2/1 -> PROCESS/1
  Sensor TF/1 -> Sum3/1
  PROPAGATION DELAY/1 -> Sum1/2  "TAU_P"
  Variable Time Delay/1 -> ACTUATOR/1
  Sum4/1 -> error/1
  Constant3/1 -> Sum4/2
  DISTURBANCE/1 -> Sum2/2
  Sum/1 -> CONTROLLER/1

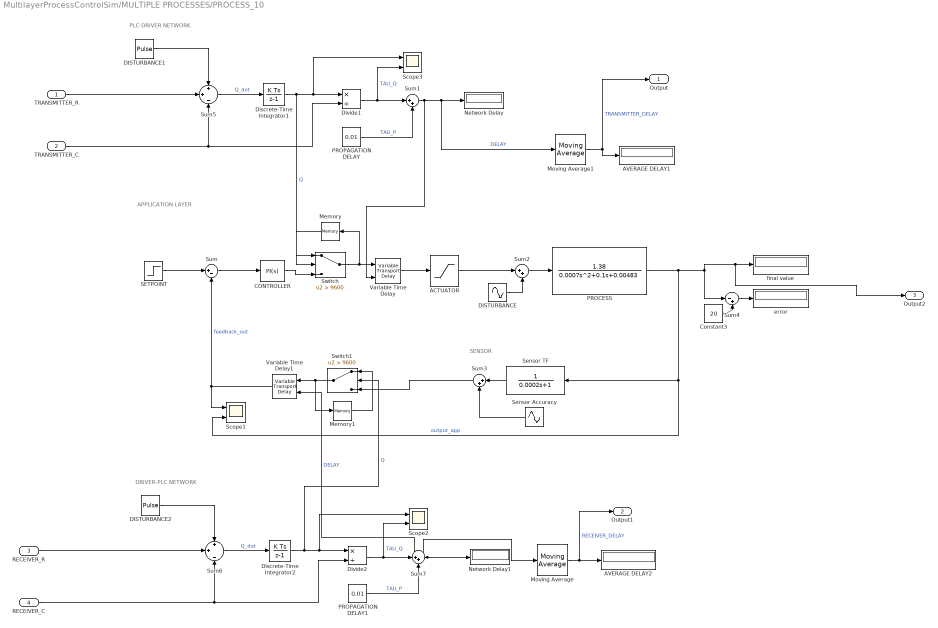
== system MultilayerProcessControlSim/MULTIPLE PROCESSES/PROCESS_10 ==
  note: DRIVER-PLC NETWORK
  note: PLC-DRIVER NETWORK
  note: APPLICATION LAYER
  note: SENSOR
  TRANSMITTER_R : Inport
  TRANSMITTER_C : Inport  Port=2
  RECEIVER_R : Inport  Port=3
  RECEIVER_C : Inport  Port=4
  ACTUATOR : Saturate  UpperLimit=150  LowerLimit=-150
  AVERAGE DELAY1 : Display
  AVERAGE DELAY2 : Display
  CONTROLLER : slpidlib/PID Controller  Controller=PI  Form=Parallel  TimeDomain=Continuous-time  UseExternalTs=off  SampleTime=-1  IntegratorMethod=Forward Euler  FilterMethod=Forward Euler  ControllerParametersSource=internal  P=1  I=3.6  UseKiTs=off  D=0  N=100  UseFilter=on  TunerSelectOption=Transfer Function Based (PID Tuner App)  InitialConditionSource=internal  InitialConditionForIntegrator=0  InitialConditionForFilter=0  DifferentiatorICPrevScaledInput=0  ExternalReset=none  TrackingMode=off  Kt=1  LimitOutput=off  SatLimitsSource=internal  UpperSaturationLimit=inf  LowerSaturationLimit=-inf  LinearizeAsGain=on  AntiWindupMode=none  Kb=1  LimitIntegrator=off  UpperIntegratorSaturationLimit=inf  LowerIntegratorSaturationLimit=-inf  POutMin=[]  POutMax=[]  IOutMin=[]  IOutMax=[]  DOutMin=[]  DOutMax=[]  NOutMin=[]  NOutMax=[]  SumOutMin=[]  SumOutMax=[]  SaturationOutMin=[]  SaturationOutMax=[]  PParamMin=[]  PParamMax=[]  IParamMin=[]  IParamMax=[]  DParamMin=[]  DParamMax=[]  NParamMin=[]  NParamMax=[]  KbParamMin=[]  KbParamMax=[]  KtParamMin=[]  KtParamMax=[]  KbOutMin=[]  KbOutMax=[]  KtOutMin=[]  KtOutMax=[]  IntegratorOutMin=[]  IntegratorOutMax=[]  FilterOutMin=[]  FilterOutMax=[]  SumI1OutMin=[]  SumI1OutMax=[]  SumI2OutMin=[]  SumI2OutMax=[]  SumI3OutMin=[]  SumI3OutMax=[]  SumI4OutMin=[]  SumI4OutMax=[]  SumDOutMin=[]  SumDOutMax=[]  DifferentiatorOutMin=[]  DifferentiatorOutMax=[]  FilterDiffOutCoefMin=[]  FilterDiffOutCoefMax=[]  ReciprocalOutMin=[]  ReciprocalOutMax=[]  SumDenOutMin=[]  SumDenOutMax=[]  SumNumOutMin=[]  SumNumOutMax=[]  DivideOutMin=[]  DivideOutMax=[]  UdiffTsProdOutMin=[]  UdiffTsProdOutMax=[]  NTsProdOutMin=[]  NTsProdOutMax=[]  UintegralTsProdOutMin=[]  UintegralTsProdOutMax=[]  UngainTsProdOutMin=[]  UngainTsProdOutMax=[]  ClampingZeroOutDataTypeStr=Inherit: Inherit via back propagation  ClampingZeroOutMin=[]  ClampingZeroOutMax=[]  FilterDenConstantOutDataTypeStr=Inherit: Inherit via back propagation  FilterDenConstantOutMin=[]  FilterDenConstantOutMax=[]  PCopyOutDataTypeStr=Inherit: Inherit via back propagation  PCopyOutMin=[]  PCopyOutMax=[]  NCopyOutDataTypeStr=Inherit: Inherit via back propagation  NCopyOutMin=[]  NCopyOutMax=[]  IntegratorContinuousStateAttributes=''  IntegratorStateMustResolveToSignalObject=off  IntegratorRTWStateStorageClass=Auto  FilterContinuousStateAttributes=''  FilterStateMustResolveToSignalObject=off  FilterRTWStateStorageClass=Auto  ParallelPVariant=InternalParameters  IdealPVariant=Disabled  IVariant=InternalParameters  DVariant=Disabled  IntegratorVariant=Continuous  SatVariant=Disabled  AWVariant=Passthrough  PCopyVariant=Disabled  TRVariant=Disabled  FdbkBlocksVariant=Forward  IdealPFdbkVariant=Disabled  SatFdbkVariant=Disabled  DerivativeFilterVariant=Disabled  NVariant=Disabled  NCopyVariant=Disabled_SignalSpec  FilterICVariant=Disabled  IntegratorICVariant=InternalICs  ExternalResetVariant=Disabled  TRSumVariant=Passthrough  SumFdbkVariant=Disabled  SumVariant=Sum_PI  TsampFilterVariant=InternalTs  TsampNgainVariant=Passthrough  TsampIntegralVariant=Disabled_SignalSpec  ExternalSaturationOutDataTypeStr=Inherit: Same as second input
  Constant3 : Constant  Value=20
  DISTURBANCE : Sin  Amplitude=0.1  Bias=0.05  Frequency=50  SampleTime=0
  DISTURBANCE1 : DiscretePulseGenerator  PulseType=Time based  Amplitude=48  Period=0.001  PulseWidth=50
  DISTURBANCE2 : DiscretePulseGenerator  PulseType=Time based  Amplitude=48  Period=0.001  PulseWidth=50
  Discrete-Time Integrator1 : DiscreteIntegrator  SampleTime=-1  LimitOutput=on  UpperSaturationLimit=9600  LowerSaturationLimit=0  ICPrevOutput=DiscIntNeverNeededParam  ICPrevScaledInput=DiscIntNeverNeededParam
  Discrete-Time Integrator2 : DiscreteIntegrator  SampleTime=-1  LimitOutput=on  UpperSaturationLimit=9600  LowerSaturationLimit=0  ICPrevOutput=DiscIntNeverNeededParam  ICPrevScaledInput=DiscIntNeverNeededParam
  Divide1 : Product  Inputs=*/
  Divide2 : Product  Inputs=*/
  Memory : Memory
  Memory1 : Memory
  Moving Average : dspstat3/Moving Average  Method=Sliding window  ForgettingFactorPort=off  SpecifyWindowLength=on  WindowLength=4  OverlapLength=3  AllowArbitraryInputLength=off  ForgettingFactor=0.9  SimulateUsing=Code generation
  Moving Average1 : dspstat3/Moving Average  Method=Sliding window  ForgettingFactorPort=off  SpecifyWindowLength=on  WindowLength=4  OverlapLength=3  AllowArbitraryInputLength=off  ForgettingFactor=0.9  SimulateUsing=Code generation
  Network Delay : Display
  Network Delay1 : Display
  PROCESS : TransferFcn  Numerator=[1.38]  Denominator=[0.0007 0.1 0.00483]
  PROPAGATION DELAY : Constant  Value=0.01
  PROPAGATION DELAY1 : Constant  Value=0.01
  SETPOINT : Step  After=20  SampleTime=0
  Scope1 : Scope  NumInputPorts=2
  Scope2 : Scope  NumInputPorts=2
  Scope3 : Scope  NumInputPorts=2
  Sensor Accuracy : Sin  Amplitude=0.01  Frequency=50  SampleTime=0
  Sensor TF : TransferFcn  Denominator=[0.0002 1]
  Sum : Sum  Inputs=|+-
  Sum{1..3,7} (4 alike) : Sum  Inputs=|++
  Sum4 : Sum  Inputs=|-+
  Sum5 : Sum  Inputs=+|+|-
  Sum6 : Sum  Inputs=+|+|-
  Switch : Switch  Criteria=u2 > Threshold  Threshold=9600  SaturateOnIntegerOverflow=off  InputSameDT=off
  Switch1 : Switch  Criteria=u2 > Threshold  Threshold=9600  SaturateOnIntegerOverflow=off  InputSameDT=off
  Variable Time Delay : VariableTransportDelay  MaximumDelay=10
  Variable Time Delay1 : VariableTransportDelay  MaximumDelay=10
  error : Display
  final value : Display
  Output : Outport
  Output1 : Outport  Port=2
  Output2 : Outport  Port=3
  wires:
  RECEIVER_C/1 -> Sum6/3, Divide2/2
  DISTURBANCE1/1 -> Sum5/1
  Sum1/1 -> Moving Average1/1, Network Delay/1, Variable Time Delay/2  "DELAY"
  TRANSMITTER_C/1 -> Divide1/2, Sum5/3
  CONTROLLER/1 -> Switch/3
  Sum3/1 -> Switch1/3
  Moving Average1/1 -> Output/1, AVERAGE DELAY1/1  "TRANSMITTER_DELAY"
  Memory1/1 -> Switch1/1
  Memory/1 -> Switch/1
  Switch/1 -> Memory/1, Variable Time Delay/1
  TRANSMITTER_R/1 -> Sum5/2
  ACTUATOR/1 -> Sum2/1
  RECEIVER_R/1 -> Sum6/2
  SETPOINT/1 -> Sum/1
  Sum7/1 -> Variable Time Delay1/2, Moving Average/1, Network Delay1/1  "DELAY"
  Discrete-Time Integrator2/1 -> Switch1/2, Scope2/1, Divide2/1  "Q"
  Switch1/1 -> Memory1/1, Variable Time Delay1/1
  DISTURBANCE2/1 -> Sum6/1
  Variable Time Delay1/1 -> Sum/2, Scope1/1  "feedback_out"
  Discrete-Time Integrator1/1 -> Scope3/1, Divide1/1, Switch/2  "Q"
  Divide2/1 -> Sum7/1, Scope2/2  "TAU_Q"
  Moving Average/1 -> Output1/1, AVERAGE DELAY2/1  "RECEIVER_DELAY"
  Divide1/1 -> Scope3/2, Sum1/1  "TAU_Q"
  Sensor Accuracy/1 -> Sum3/2
  Sum6/1 -> Discrete-Time Integrator2/1  "Q_dot"
  PROCESS/1 -> Output2/1, final value/1, Sum4/1, Sensor TF/1, Scope1/2  "output_app"
  PROPAGATION DELAY1/1 -> Sum7/2  "TAU_P"
  Sum5/1 -> Discrete-Time Integrator1/1  "Q_dot"
  Sum2/1 -> PROCESS/1
  Sensor TF/1 -> Sum3/1
  PROPAGATION DELAY/1 -> Sum1/2  "TAU_P"
  Variable Time Delay/1 -> ACTUATOR/1
  Sum4/1 -> error/1
  Constant3/1 -> Sum4/2
  DISTURBANCE/1 -> Sum2/2
  Sum/1 -> CONTROLLER/1

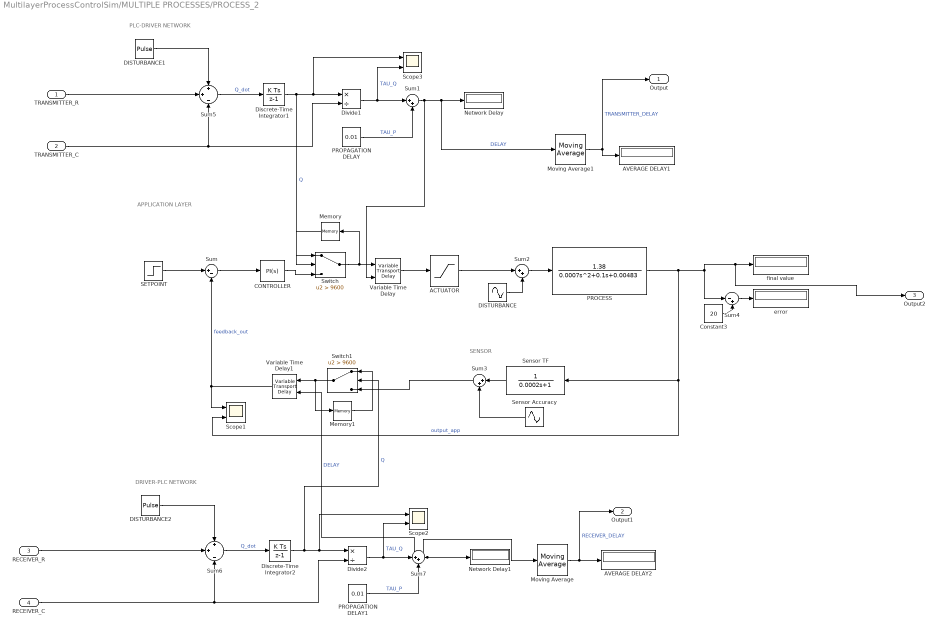
== system MultilayerProcessControlSim/MULTIPLE PROCESSES/PROCESS_2 ==
  note: SENSOR
  note: APPLICATION LAYER
  note: PLC-DRIVER NETWORK
  note: DRIVER-PLC NETWORK
  TRANSMITTER_R : Inport
  TRANSMITTER_C : Inport  Port=2
  RECEIVER_R : Inport  Port=3
  RECEIVER_C : Inport  Port=4
  ACTUATOR : Saturate  UpperLimit=150  LowerLimit=-150
  AVERAGE DELAY1 : Display
  AVERAGE DELAY2 : Display
  CONTROLLER : slpidlib/PID Controller  Controller=PI  Form=Parallel  TimeDomain=Continuous-time  UseExternalTs=off  SampleTime=-1  IntegratorMethod=Forward Euler  FilterMethod=Forward Euler  ControllerParametersSource=internal  P=1  I=3.6  UseKiTs=off  D=0  N=100  UseFilter=on  TunerSelectOption=Transfer Function Based (PID Tuner App)  InitialConditionSource=internal  InitialConditionForIntegrator=0  InitialConditionForFilter=0  DifferentiatorICPrevScaledInput=0  ExternalReset=none  TrackingMode=off  Kt=1  LimitOutput=off  SatLimitsSource=internal  UpperSaturationLimit=inf  LowerSaturationLimit=-inf  LinearizeAsGain=on  AntiWindupMode=none  Kb=1  LimitIntegrator=off  UpperIntegratorSaturationLimit=inf  LowerIntegratorSaturationLimit=-inf  POutMin=[]  POutMax=[]  IOutMin=[]  IOutMax=[]  DOutMin=[]  DOutMax=[]  NOutMin=[]  NOutMax=[]  SumOutMin=[]  SumOutMax=[]  SaturationOutMin=[]  SaturationOutMax=[]  PParamMin=[]  PParamMax=[]  IParamMin=[]  IParamMax=[]  DParamMin=[]  DParamMax=[]  NParamMin=[]  NParamMax=[]  KbParamMin=[]  KbParamMax=[]  KtParamMin=[]  KtParamMax=[]  KbOutMin=[]  KbOutMax=[]  KtOutMin=[]  KtOutMax=[]  IntegratorOutMin=[]  IntegratorOutMax=[]  FilterOutMin=[]  FilterOutMax=[]  SumI1OutMin=[]  SumI1OutMax=[]  SumI2OutMin=[]  SumI2OutMax=[]  SumI3OutMin=[]  SumI3OutMax=[]  SumI4OutMin=[]  SumI4OutMax=[]  SumDOutMin=[]  SumDOutMax=[]  DifferentiatorOutMin=[]  DifferentiatorOutMax=[]  FilterDiffOutCoefMin=[]  FilterDiffOutCoefMax=[]  ReciprocalOutMin=[]  ReciprocalOutMax=[]  SumDenOutMin=[]  SumDenOutMax=[]  SumNumOutMin=[]  SumNumOutMax=[]  DivideOutMin=[]  DivideOutMax=[]  UdiffTsProdOutMin=[]  UdiffTsProdOutMax=[]  NTsProdOutMin=[]  NTsProdOutMax=[]  UintegralTsProdOutMin=[]  UintegralTsProdOutMax=[]  UngainTsProdOutMin=[]  UngainTsProdOutMax=[]  ClampingZeroOutDataTypeStr=Inherit: Inherit via back propagation  ClampingZeroOutMin=[]  ClampingZeroOutMax=[]  FilterDenConstantOutDataTypeStr=Inherit: Inherit via back propagation  FilterDenConstantOutMin=[]  FilterDenConstantOutMax=[]  PCopyOutDataTypeStr=Inherit: Inherit via back propagation  PCopyOutMin=[]  PCopyOutMax=[]  NCopyOutDataTypeStr=Inherit: Inherit via back propagation  NCopyOutMin=[]  NCopyOutMax=[]  IntegratorContinuousStateAttributes=''  IntegratorStateMustResolveToSignalObject=off  IntegratorRTWStateStorageClass=Auto  FilterContinuousStateAttributes=''  FilterStateMustResolveToSignalObject=off  FilterRTWStateStorageClass=Auto  ParallelPVariant=InternalParameters  IdealPVariant=Disabled  IVariant=InternalParameters  DVariant=Disabled  IntegratorVariant=Continuous  SatVariant=Disabled  AWVariant=Passthrough  PCopyVariant=Disabled  TRVariant=Disabled  FdbkBlocksVariant=Forward  IdealPFdbkVariant=Disabled  SatFdbkVariant=Disabled  DerivativeFilterVariant=Disabled  NVariant=Disabled  NCopyVariant=Disabled_SignalSpec  FilterICVariant=Disabled  IntegratorICVariant=InternalICs  ExternalResetVariant=Disabled  TRSumVariant=Passthrough  SumFdbkVariant=Disabled  SumVariant=Sum_PI  TsampFilterVariant=InternalTs  TsampNgainVariant=Passthrough  TsampIntegralVariant=Disabled_SignalSpec  ExternalSaturationOutDataTypeStr=Inherit: Same as second input
  Constant3 : Constant  Value=20
  DISTURBANCE : Sin  Amplitude=0.1  Bias=0.05  Frequency=50  SampleTime=0
  DISTURBANCE1 : DiscretePulseGenerator  PulseType=Time based  Amplitude=16  Period=1  PulseWidth=50
  DISTURBANCE2 : DiscretePulseGenerator  PulseType=Time based  Amplitude=16  Period=1  PulseWidth=50
  Discrete-Time Integrator1 : DiscreteIntegrator  SampleTime=-1  LimitOutput=on  UpperSaturationLimit=9600  LowerSaturationLimit=0  ICPrevOutput=DiscIntNeverNeededParam  ICPrevScaledInput=DiscIntNeverNeededParam
  Discrete-Time Integrator2 : DiscreteIntegrator  SampleTime=-1  LimitOutput=on  UpperSaturationLimit=9600  LowerSaturationLimit=0  ICPrevOutput=DiscIntNeverNeededParam  ICPrevScaledInput=DiscIntNeverNeededParam
  Divide1 : Product  Inputs=*/
  Divide2 : Product  Inputs=*/
  Memory : Memory
  Memory1 : Memory
  Moving Average : dspstat3/Moving Average  Method=Sliding window  ForgettingFactorPort=off  SpecifyWindowLength=on  WindowLength=4  OverlapLength=3  AllowArbitraryInputLength=off  ForgettingFactor=0.9  SimulateUsing=Code generation
  Moving Average1 : dspstat3/Moving Average  Method=Sliding window  ForgettingFactorPort=off  SpecifyWindowLength=on  WindowLength=4  OverlapLength=3  AllowArbitraryInputLength=off  ForgettingFactor=0.9  SimulateUsing=Code generation
  Network Delay : Display
  Network Delay1 : Display
  PROCESS : TransferFcn  Numerator=[1.38]  Denominator=[0.0007 0.1 0.00483]
  PROPAGATION DELAY : Constant  Value=0.01
  PROPAGATION DELAY1 : Constant  Value=0.01
  SETPOINT : Step  After=20  SampleTime=0
  Scope1 : Scope  NumInputPorts=2
  Scope2 : Scope  NumInputPorts=2
  Scope3 : Scope  NumInputPorts=2
  Sensor Accuracy : Sin  Amplitude=0.01  Frequency=50  SampleTime=0
  Sensor TF : TransferFcn  Denominator=[0.0002 1]
  Sum : Sum  Inputs=|+-
  Sum{1..3,7} (4 alike) : Sum  Inputs=|++
  Sum4 : Sum  Inputs=|-+
  Sum5 : Sum  Inputs=+|+|-
  Sum6 : Sum  Inputs=+|+|-
  Switch : Switch  Criteria=u2 > Threshold  Threshold=9600  SaturateOnIntegerOverflow=off  InputSameDT=off
  Switch1 : Switch  Criteria=u2 > Threshold  Threshold=9600  SaturateOnIntegerOverflow=off  InputSameDT=off
  Variable Time Delay : VariableTransportDelay  MaximumDelay=10
  Variable Time Delay1 : VariableTransportDelay  MaximumDelay=10
  error : Display
  final value : Display
  Output : Outport
  Output1 : Outport  Port=2
  Output2 : Outport  Port=3
  wires:
  Sum/1 -> CONTROLLER/1
  DISTURBANCE/1 -> Sum2/2
  Constant3/1 -> Sum4/2
  Sum4/1 -> error/1
  Variable Time Delay/1 -> ACTUATOR/1
  PROPAGATION DELAY/1 -> Sum1/2  "TAU_P"
  Sensor TF/1 -> Sum3/1
  Sum2/1 -> PROCESS/1
  Sum5/1 -> Discrete-Time Integrator1/1  "Q_dot"
  PROPAGATION DELAY1/1 -> Sum7/2  "TAU_P"
  PROCESS/1 -> Scope1/2, Sensor TF/1, Sum4/1, final value/1, Output2/1  "output_app"
  Sum6/1 -> Discrete-Time Integrator2/1  "Q_dot"
  Sensor Accuracy/1 -> Sum3/2
  Divide1/1 -> Sum1/1, Scope3/2  "TAU_Q"
  Moving Average/1 -> AVERAGE DELAY2/1, Output1/1  "RECEIVER_DELAY"
  Divide2/1 -> Scope2/2, Sum7/1  "TAU_Q"
  Discrete-Time Integrator1/1 -> Switch/2, Divide1/1, Scope3/1  "Q"
  Variable Time Delay1/1 -> Scope1/1, Sum/2  "feedback_out"
  DISTURBANCE2/1 -> Sum6/1
  Switch1/1 -> Variable Time Delay1/1, Memory1/1
  Discrete-Time Integrator2/1 -> Divide2/1, Scope2/1, Switch1/2  "Q"
  Sum7/1 -> Network Delay1/1, Moving Average/1, Variable Time Delay1/2  "DELAY"
  SETPOINT/1 -> Sum/1
  RECEIVER_R/1 -> Sum6/2
  ACTUATOR/1 -> Sum2/1
  TRANSMITTER_R/1 -> Sum5/2
  Switch/1 -> Variable Time Delay/1, Memory/1
  Memory/1 -> Switch/1
  Memory1/1 -> Switch1/1
  Moving Average1/1 -> AVERAGE DELAY1/1, Output/1  "TRANSMITTER_DELAY"
  Sum3/1 -> Switch1/3
  CONTROLLER/1 -> Switch/3
  TRANSMITTER_C/1 -> Sum5/3, Divide1/2
  Sum1/1 -> Variable Time Delay/2, Network Delay/1, Moving Average1/1  "DELAY"
  DISTURBANCE1/1 -> Sum5/1
  RECEIVER_C/1 -> Divide2/2, Sum6/3
